simulink model "activeBalancing2"  (R2021a)
settings: Solver=VariableStepAuto  StartTime=0.0  StopTime=120  RelTol=1e-3
undefined symbols (not defined in the file): Ion, Lithium
libraries: spsSeriesRLCBranchLib x16, spsMosfetLib x14, simulink x9, spsBatteryLib x7, fuzblock x6, spspowerguiLib x1
settings Model: SimulationMode=rapid-accelerator  PacingRate=1000  Creator=Navadeep  LastModifiedBy=Navadeep

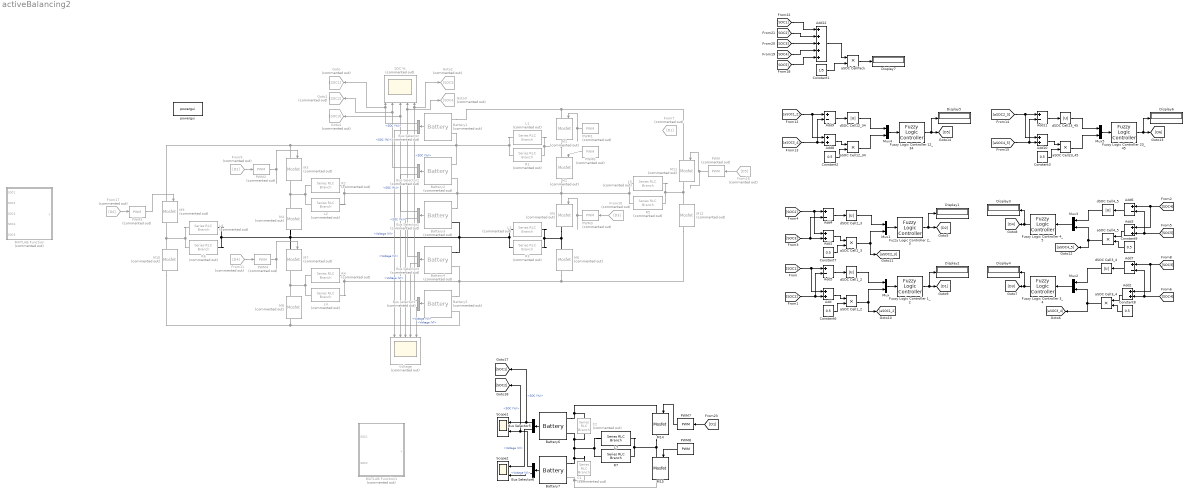
== system activeBalancing2 ==
  Add{,1..3,8,10} (6 alike) : Sum
  Add{4..7,9,11} (6 alike) : Sum  Inputs=+-
  Add12 : Sum  Inputs=+++++
  Battery1 : spsBatteryLib/Battery  Commented=on  BatType=Lithium-Ion  ShowTempParam=off  ThermalPreset=no  ShowAgeParam=off  NomV=3.7  NomQ=6  SOC=85  Batt_Tr=30  PresetModel=on  MaxQ=6  MinV=2.775  FullV=4.3068  Dis_rate=2.6087  R=0.0061667  Normal_OP=5.4261  expZone="[3.9974     0.29478]"  current=[6.5 13 32.5]  Units=Time  Tci=20  NomT=20  T2=-30  MaxQ2=4.8  FullV2=7.1  Normal_OP2=5.655  expZone2="[6.58           1]"  Rca=0.6  ti=2000  Dp=0  Neq0=0  Tsim=1e6  Ta1=25  Qeol=5.4*0.9  Reol=0.013333*1.2  Char_age=[2.3478, 3]  Dis_age=[2.3478, 10]  N1=1500  N2=10500  N3=1000  N4=1400  Ta2=45  N5=950
  Battery2 : spsBatteryLib/Battery  Commented=on  BatType=Lithium-Ion  ShowTempParam=off  ThermalPreset=no  ShowAgeParam=off  NomV=3.7  NomQ=6  SOC=82  Batt_Tr=30  PresetModel=on  MaxQ=6  MinV=2.775  FullV=4.3068  Dis_rate=2.6087  R=0.0061667  Normal_OP=5.4261  expZone="[3.9974     0.29478]"  current=[6.5 13 32.5]  Units=Time  Tci=20  NomT=20  T2=-30  MaxQ2=4.8  FullV2=7.1  Normal_OP2=5.655  expZone2="[6.58           1]"  Rca=0.6  ti=2000  Dp=0  Neq0=0  Tsim=1e6  Ta1=25  Qeol=5.4*0.9  Reol=0.013333*1.2  Char_age=[2.3478, 3]  Dis_age=[2.3478, 10]  N1=1500  N2=10500  N3=1000  N4=1400  Ta2=45  N5=950
  Battery3 : spsBatteryLib/Battery  Commented=on  BatType=Lithium-Ion  ShowTempParam=off  ThermalPreset=no  ShowAgeParam=off  NomV=3.7  NomQ=6  SOC=84  Batt_Tr=30  PresetModel=on  MaxQ=6  MinV=2.775  FullV=4.3068  Dis_rate=2.6087  R=0.0061667  Normal_OP=5.4261  expZone="[3.9974     0.29478]"  current=[6.5 13 32.5]  Units=Time  Tci=20  NomT=20  T2=-30  MaxQ2=4.8  FullV2=7.1  Normal_OP2=5.655  expZone2="[6.58           1]"  Rca=0.6  ti=2000  Dp=0  Neq0=0  Tsim=1e6  Ta1=25  Qeol=5.4*0.9  Reol=0.013333*1.2  Char_age=[2.3478, 3]  Dis_age=[2.3478, 10]  N1=1500  N2=10500  N3=1000  N4=1400  Ta2=45  N5=950
  Battery4 : spsBatteryLib/Battery  Commented=on  BatType=Lithium-Ion  ShowTempParam=off  ThermalPreset=no  ShowAgeParam=off  NomV=3.7  NomQ=6  SOC=81  Batt_Tr=30  PresetModel=on  MaxQ=6  MinV=2.775  FullV=4.3068  Dis_rate=2.6087  R=0.0061667  Normal_OP=5.4261  expZone="[3.9974     0.29478]"  current=[6.5 13 32.5]  Units=Time  Tci=20  NomT=20  T2=-30  MaxQ2=4.8  FullV2=7.1  Normal_OP2=5.655  expZone2="[6.58           1]"  Rca=0.6  ti=2000  Dp=0  Neq0=0  Tsim=1e6  Ta1=25  Qeol=5.4*0.9  Reol=0.013333*1.2  Char_age=[2.3478, 3]  Dis_age=[2.3478, 10]  N1=1500  N2=10500  N3=1000  N4=1400  Ta2=45  N5=950
  Battery5 : spsBatteryLib/Battery  Commented=on  BatType=Lithium-Ion  ShowTempParam=off  ThermalPreset=no  ShowAgeParam=off  NomV=3.7  NomQ=6  SOC=83  Batt_Tr=30  PresetModel=on  MaxQ=6  MinV=2.775  FullV=4.3068  Dis_rate=2.6087  R=0.0061667  Normal_OP=5.4261  expZone="[3.9974     0.29478]"  current=[6.5 13 32.5]  Units=Time  Tci=20  NomT=20  T2=-30  MaxQ2=4.8  FullV2=7.1  Normal_OP2=5.655  expZone2="[6.58           1]"  Rca=0.6  ti=2000  Dp=0  Neq0=0  Tsim=1e6  Ta1=25  Qeol=5.4*0.9  Reol=0.013333*1.2  Char_age=[2.3478, 3]  Dis_age=[2.3478, 10]  N1=1500  N2=10500  N3=1000  N4=1400  Ta2=45  N5=950
  Battery6 : spsBatteryLib/Battery  BatType=Lithium-Ion  ShowTempParam=off  ThermalPreset=no  ShowAgeParam=off  NomV=3.7  NomQ=6  SOC=75  Batt_Tr=30  PresetModel=on  MaxQ=6  MinV=2.775  FullV=4.3068  Dis_rate=2.6087  R=0.0061667  Normal_OP=5.4261  expZone="[3.9974     0.29478]"  current=[6.5 13 32.5]  Units=Time  Tci=20  NomT=20  T2=-30  MaxQ2=4.8  FullV2=7.1  Normal_OP2=5.655  expZone2="[6.58           1]"  Rca=0.6  ti=2000  Dp=0  Neq0=0  Tsim=1e6  Ta1=25  Qeol=5.4*0.9  Reol=0.013333*1.2  Char_age=[2.3478, 3]  Dis_age=[2.3478, 10]  N1=1500  N2=10500  N3=1000  N4=1400  Ta2=45  N5=950
  Battery7 : spsBatteryLib/Battery  BatType=Lithium-Ion  ShowTempParam=off  ThermalPreset=no  ShowAgeParam=off  NomV=3.7  NomQ=6  SOC=80  Batt_Tr=30  PresetModel=on  MaxQ=6  MinV=2.775  FullV=4.3068  Dis_rate=2.6087  R=0.0061667  Normal_OP=5.4261  expZone="[3.9974     0.29478]"  current=[6.5 13 32.5]  Units=Time  Tci=20  NomT=20  T2=-30  MaxQ2=4.8  FullV2=7.1  Normal_OP2=5.655  expZone2="[6.58           1]"  Rca=0.6  ti=2000  Dp=0  Neq0=0  Tsim=1e6  Ta1=25  Qeol=5.4*0.9  Reol=0.013333*1.2  Char_age=[2.3478, 3]  Dis_age=[2.3478, 10]  N1=1500  N2=10500  N3=1000  N4=1400  Ta2=45  N5=950
  Bus Selector{,1..4} (5 alike) : BusSelector  Commented=on  OutputSignals=SOC (%),Voltage (V)
  Bus Selector5 : BusSelector  OutputSignals=SOC (%),Voltage (V)
  Bus Selector6 : BusSelector  OutputSignals=SOC (%),Voltage (V)
  C1 : spsSeriesRLCBranchLib/Series RLC Branch  Commented=on  LConnTagsString=__new0  RConnTagsString=__new0  BranchType=C  Resistance=1  Inductance=1e-3  SetiL0=off  InitialCurrent=0  Capacitance=22e-6  Setx0=off  InitialVoltage=0  Measurements=None
  C2 : spsSeriesRLCBranchLib/Series RLC Branch  Commented=on  LConnTagsString=__new0  RConnTagsString=__new0  BranchType=C  Resistance=1  Inductance=1e-3  SetiL0=off  InitialCurrent=0  Capacitance=22e-6  Setx0=off  InitialVoltage=0  Measurements=None
  Constant1 : Constant  Value=1/5
  Constant{2..3,6..9} (6 alike) : Constant  Value=0.5
  Display{1..7} (7 alike) : Display
  From10 : From  Commented=on  GotoTag=D3
  From11 : From  Commented=on  GotoTag=D4
  From16 : From  Commented=on  GotoTag=D5
  From17 : From  Commented=on  GotoTag=D6
  From7 : From  Commented=on  GotoTag=D1
  From9 : From  Commented=on  GotoTag=D2
  Fuzzy Logic Controller 12_34 : fuzblock/Fuzzy Logic  Controller  FIS='cell12_34.fis'  OutputSampleNumber=101  DataType=double  FuzzifiedInputs=off  RuleFiringStrengths=off  RuleOutputs=off  AggregatedOutputs=off  SimulateUsing=Interpreted execution  OutOfRangeInputValueMessage=warning  NoRuleFiredMessage=warning  EmptyOutputFuzzySetMessage=warning
  Fuzzy Logic Controller 1_2 : fuzblock/Fuzzy Logic  Controller  FIS='cell1_2.fis'  OutputSampleNumber=101  DataType=double  FuzzifiedInputs=off  RuleFiringStrengths=off  RuleOutputs=off  AggregatedOutputs=off  SimulateUsing=Interpreted execution  OutOfRangeInputValueMessage=warning  NoRuleFiredMessage=warning  EmptyOutputFuzzySetMessage=warning
  Fuzzy Logic Controller 23_45 : fuzblock/Fuzzy Logic  Controller  FIS='cell23_45.fis'  OutputSampleNumber=101  DataType=double  FuzzifiedInputs=off  RuleFiringStrengths=off  RuleOutputs=off  AggregatedOutputs=off  SimulateUsing=Interpreted execution  OutOfRangeInputValueMessage=warning  NoRuleFiredMessage=warning  EmptyOutputFuzzySetMessage=warning
  Fuzzy Logic Controller 2_3 : fuzblock/Fuzzy Logic  Controller  FIS='cell2_3.fis'  OutputSampleNumber=101  DataType=double  FuzzifiedInputs=off  RuleFiringStrengths=off  RuleOutputs=off  AggregatedOutputs=off  SimulateUsing=Interpreted execution  OutOfRangeInputValueMessage=warning  NoRuleFiredMessage=warning  EmptyOutputFuzzySetMessage=warning
  Fuzzy Logic Controller 3_4 : fuzblock/Fuzzy Logic  Controller  FIS='cell3_4.fis'  OutputSampleNumber=101  DataType=double  FuzzifiedInputs=off  RuleFiringStrengths=off  RuleOutputs=off  AggregatedOutputs=off  SimulateUsing=Interpreted execution  OutOfRangeInputValueMessage=warning  NoRuleFiredMessage=warning  EmptyOutputFuzzySetMessage=warning
  Fuzzy Logic Controller 4_5 : fuzblock/Fuzzy Logic  Controller  FIS='cell4_5.fis'  OutputSampleNumber=101  DataType=double  FuzzifiedInputs=off  RuleFiringStrengths=off  RuleOutputs=off  AggregatedOutputs=off  SimulateUsing=Interpreted execution  OutOfRangeInputValueMessage=warning  NoRuleFiredMessage=warning  EmptyOutputFuzzySetMessage=warning
  Goto : Goto  Commented=on  GotoTag=SOC1
  Goto1 : Goto  Commented=on  GotoTag=SOC2
  Goto2 : Goto  Commented=on  GotoTag=SOC5
  Goto3 : Goto  Commented=on  GotoTag=SOC4
  Goto4 : Goto  Commented=on  GotoTag=SOC3
  L{1..6} (6 alike) : spsSeriesRLCBranchLib/Series RLC Branch  Commented=on  LConnTagsString=__new0  RConnTagsString=__new0  BranchType=L  Resistance=1  Inductance=56e-6  SetiL0=off  InitialCurrent=0  Capacitance=1e-6  Setx0=off  InitialVoltage=0  Measurements=None
  L7 : spsSeriesRLCBranchLib/Series RLC Branch  LConnTagsString=__new0  RConnTagsString=__new0  BranchType=L  Resistance=1  Inductance=56e-6  SetiL0=off  InitialCurrent=0  Capacitance=1e-6  Setx0=off  InitialVoltage=0  Measurements=None
  M{1..12} (12 alike) : spsMosfetLib/Mosfet  Commented=on  Ron=0.1  Lon=0  Rd=0.01  Vfd=0  IC=0  Rs=1e5  Cs=inf  Measurements=on
  M14 : spsMosfetLib/Mosfet  Ron=0.1  Lon=0  Rd=0.01  Vfd=0  IC=0  Rs=1e5  Cs=inf  Measurements=on
  M15 : spsMosfetLib/Mosfet  Ron=0.1  Lon=0  Rd=0.01  Vfd=0  IC=0  Rs=1e5  Cs=inf  Measurements=on
  MATLAB Function : MATLAB Function  Commented=on  TreatAsAtomicUnit=on
  MATLAB Function1 : MATLAB Function  Commented=on  TreatAsAtomicUnit=on
  Mux{,1..5} (6 alike) : Mux  Inputs=2
  PWM{,1..6} (7 alike) : simulink/Discontinuities/PWM  Commented=on  DisableCoverage=on  Period=1e-3  DisallowZeroDutyCycle=off  RunAtFixedTimeIntervals=off  SampleTime=0.1
  PWM7 : simulink/Discontinuities/PWM  DisableCoverage=on  Period=1e-3  DisallowZeroDutyCycle=off  RunAtFixedTimeIntervals=off  SampleTime=0.1
  PWM8 : simulink/Discontinuities/PWM  DisableCoverage=on  Period=1e-3  DisallowZeroDutyCycle=off  RunAtFixedTimeIntervals=off  SampleTime=0.1
  R{1..6} (6 alike) : spsSeriesRLCBranchLib/Series RLC Branch  Commented=on  LConnTagsString=__new0  RConnTagsString=__new0  BranchType=R  Resistance=2000  Inductance=1e-3  SetiL0=off  InitialCurrent=0  Capacitance=1e-6  Setx0=off  InitialVoltage=0  Measurements=None
  R7 : spsSeriesRLCBranchLib/Series RLC Branch  LConnTagsString=__new0  RConnTagsString=__new0  BranchType=R  Resistance=2000  Inductance=1e-3  SetiL0=off  InitialCurrent=0  Capacitance=1e-6  Setx0=off  InitialVoltage=0  Measurements=None
  SOC % : Scope  Commented=on  NumInputPorts=5
  Scope1 : Scope  NumInputPorts=2
  Scope2 : Scope  NumInputPorts=2
  Voltage : Scope  Commented=on  NumInputPorts=5
  aSOC Cell12_34 : Product
  aSOC Cell1_2 : Product
  aSOC Cell23_45 : Product
  aSOC Cell2_3 : Product
  aSOC Cell3_4 : Product
  aSOC Cell4_5 : Product
  aSOC CellPack : Product
  dSOC Cell12_34 : Abs
  dSOC Cell1_2 : Abs  ZeroCross=off
  dSOC Cell23_45 : Abs
  dSOC Cell2_3 : Abs
  dSOC Cell3_4 : Abs
  dSOC Cell4_5 : Abs
  powergui : spspowerguiLib/powergui  Priority=1  SimulationMode=Continuous  SampleTime=50e-3  frequency=60  Iterations=50  frequencyindice=0  Pbase=100e6  ErrMax=1e-4  UnitsV=kV  UnitsW=MW  buscounter=0  FunctionMessages=off  echomessages=off  EnableUseOfTLC=off  CurrentSourceSwitches=off  DisableSnubberDevices=off  DisableRonSwitches=off  DisableVfSwitches=off  DisplayEquations=off  AutomaticDiscreteSolvers=off  SolverType=Tustin/Backward Euler (TBE)  Interpol=off  ExternalGateDelay=off  methode=off  Ts=100  x0status=blocks  SPID=on  SwTol=0  HookPort=off  NonlinearTolerance=1e-4  nMaxIteration=100  ContinueOnMaxIteration=off  RestoreLinks=warning  ResistiveCurrentMeasurement=off  Frange=[0:2:500]  Ylog=off  Xlog=on  ShowGrid=off  save=off  variable=ZData  structure=0  ZoomFFT=off  StartTime=0.0  cycles=1  DisplayStyle=1  fundamental=60  FreqAxis=off  MaxFrequency=1000  frequencyindicesteady=1  RmsSteady=1  display=off
  wires:
  Battery1/1 -> Bus Selector/1
  Battery2/1 -> Bus Selector1/1
  Battery4/1 -> Bus Selector3/1
  Battery3/1 -> Bus Selector2/1
  Battery5/1 -> Bus Selector4/1
  Bus Selector/1 -> Goto/1, SOC %/1  "<SOC (%)>"
  Bus Selector/2 -> Voltage/1  "<Voltage (V)>"
  Bus Selector1/2 -> Voltage/2  "<Voltage (V)>"
  Bus Selector2/2 -> Voltage/3  "<Voltage (V)>"
  Bus Selector3/2 -> Voltage/4  "<Voltage (V)>"
  Bus Selector4/2 -> Voltage/5  "<Voltage (V)>"
  PWM1/1 -> M1/1
  PWM3/1 -> M5/1
  PWM2/1 -> M3/1
  PWM4/1 -> M7/1
  PWM5/1 -> M9/1
  PWM/1 -> M11/1
  ? -> M12/1
  ? -> M6/1
  ? -> M4/1
  ? -> M8/1
  From16/1 -> PWM/1
  From10/1 -> PWM3/1
  From9/1 -> PWM2/1
  From11/1 -> PWM4/1
  From17/1 -> PWM5/1
  Mux/1 -> Fuzzy Logic Controller 1_2/1
  Bus Selector1/1 -> SOC %/2, Goto1/1  "<SOC (%)>"
  Bus Selector2/1 -> SOC %/3, Goto4/1  "<SOC (%)>"
  Bus Selector3/1 -> SOC %/4, Goto3/1  "<SOC (%)>"
  Bus Selector4/1 -> SOC %/5, Goto2/1  "<SOC (%)>"
  dSOC Cell1_2/1 -> Mux/1
  aSOC Cell1_2/1 -> [aSOC1_2], Mux/2
  Add4/1 -> dSOC Cell2_3/1
  Add5/1 -> dSOC Cell1_2/1
  [SOC2] -> Add5/2, Add/2
  [SOC1] -> Add5/1, Add/1
  Add1/1 -> aSOC Cell2_3/1
  Constant7/1 -> aSOC Cell2_3/2
  Constant6/1 -> aSOC Cell1_2/2
  Add/1 -> aSOC Cell1_2/1
  PWM6/1 -> M2/1
  Add7/1 -> dSOC Cell3_4/1
  Add6/1 -> dSOC Cell4_5/1
  [SOC5] -> Add3/2, Add6/2
  Constant8/1 -> aSOC Cell3_4/2
  Add2/1 -> aSOC Cell3_4/1
  [SOC3] -> Add2/1, Add7/1
  [SOC4] -> Add2/2, Add7/2
  [SOC4] -> Add6/1, Add3/1
  Constant9/1 -> aSOC Cell4_5/2
  Add3/1 -> aSOC Cell4_5/1
  [SOC2] -> Add1/1, Add4/1
  [SOC3] -> Add4/2, Add1/2
  Fuzzy Logic Controller 1_2/1 -> [D1], Display2/1
  Mux3/1 -> Fuzzy Logic Controller 4_5/1
  Mux2/1 -> Fuzzy Logic Controller 3_4/1
  dSOC Cell3_4/1 -> Mux2/1
  aSOC Cell3_4/1 -> Mux2/2, [aSOC3_4]
  dSOC Cell4_5/1 -> Mux3/1
  aSOC Cell4_5/1 -> [aSOC4_5], Mux3/2
  dSOC Cell2_3/1 -> Mux1/1
  aSOC Cell2_3/1 -> [aSOC2_3], Mux1/2
  Mux1/1 -> Fuzzy Logic Controller 2_3/1
  Fuzzy Logic Controller 2_3/1 -> [D2], Display1/1
  Fuzzy Logic Controller 4_5/1 -> [D4], Display3/1
  Fuzzy Logic Controller 3_4/1 -> [D3], Display4/1
  [aSOC1_2] -> Add9/1, Add8/1
  aSOC Cell12_34/1 -> Mux4/2
  dSOC Cell12_34/1 -> Mux4/1
  Fuzzy Logic Controller 12_34/1 -> [D5], Display5/1
  Mux4/1 -> Fuzzy Logic Controller 12_34/1
  Constant2/1 -> aSOC Cell12_34/2
  [aSOC3_4] -> Add9/2, Add8/2
  Add8/1 -> aSOC Cell12_34/1
  Add9/1 -> dSOC Cell12_34/1
  Add10/1 -> aSOC Cell23_45/1
  Add11/1 -> dSOC Cell23_45/1
  Constant3/1 -> aSOC Cell23_45/2
  [aSOC2_3] -> Add11/1, Add10/1
  dSOC Cell23_45/1 -> Mux5/1
  aSOC Cell23_45/1 -> Mux5/2
  Fuzzy Logic Controller 23_45/1 -> [D6], Display6/1
  Mux5/1 -> Fuzzy Logic Controller 23_45/1
  [aSOC4_5] -> Add11/2, Add10/2
  Add12/1 -> aSOC CellPack/1
  Constant1/1 -> aSOC CellPack/2
  aSOC CellPack/1 -> Display7/1
  [SOC5] -> Add12/5
  [SOC4] -> Add12/4
  [SOC3] -> Add12/3
  [SOC1] -> Add12/1
  [SOC2] -> Add12/2
  [D1] -> PWM7/1
  PWM8/1 -> M15/1
  PWM7/1 -> M14/1
  Battery6/1 -> Bus Selector5/1
  Battery7/1 -> Bus Selector6/1
  Bus Selector5/1 -> Scope1/1, [SOC1]  "<SOC (%)>"
  Bus Selector6/2 -> Scope2/2  "<Voltage (V)>"
  Bus Selector6/1 -> [SOC2], Scope1/2  "<SOC (%)>"
  Bus Selector5/2 -> Scope2/1  "<Voltage (V)>"
  connections:
  L1/RConn1 -- M2/LConn1 -- M1/RConn1 -- R1/RConn1
  L1/LConn1 -- Battery1/LConn2 -- Battery2/LConn1 -- M9/LConn1 -- M3/LConn1 -- R1/LConn1
  Battery1/LConn1 -- M11/LConn1 -- M1/LConn1
  L5/LConn1 -- R5/LConn1 -- M2/RConn1 -- M5/LConn1 -- Battery2/LConn2 -- Battery3/LConn1 -- R2/LConn1 -- L2/LConn1
  L2/RConn1 -- M4/LConn1 -- M3/RConn1 -- R2/RConn1
  R6/RConn1 -- M7/LConn1 -- M4/RConn1 -- L3/LConn1 -- R3/LConn1 -- Battery4/LConn1 -- Battery3/LConn2 -- L6/RConn1
  R3/RConn1 -- M6/LConn1 -- M5/RConn1 -- L3/RConn1
  L4/LConn1 -- M12/RConn1 -- M6/RConn1 -- Battery5/LConn1 -- Battery4/LConn2 -- R4/LConn1
  L4/RConn1 -- M8/LConn1 -- M7/RConn1 -- R4/RConn1
  M8/RConn1 -- M10/RConn1 -- Battery5/LConn2
  M11/RConn1 -- M12/LConn1 -- L5/RConn1 -- R5/RConn1
  M10/LConn1 -- M9/RConn1 -- L6/LConn1 -- R6/LConn1
  L7/LConn1 -- R7/LConn1 -- Battery7/LConn1 -- C1/LConn1 -- C2/RConn1 -- Battery6/LConn2
  M15/LConn1 -- M14/RConn1 -- L7/RConn1 -- R7/RConn1
  Battery6/LConn1 -- C2/LConn1 -- M14/LConn1
  C1/RConn1 -- M15/RConn1 -- Battery7/LConn2

== matlab function activeBalancing2/MATLAB Function1 ==
  data: SOC1 input; y output; SOC2 input
function y = fcn(SOC1, SOC2)

end

== matlab function activeBalancing2/MATLAB Function ==
  data: SOC1 input; y output; SOC2 input; SOC3 input; SOC4 input; SOC5 input
function y = fcn(SOC1, SOC2, SOC3, SOC4, SOC5)

end
